simulink model "Speed_Controller_Test_forTD"  (Simulink 6.6)
settings: Solver=ode4  SolverMode=SingleTasking  StartTime=0.0  StopTime=252  FixedStep=0.01  RelTol=1e-3
InitFcn:
  | tempomat_para
StopFcn:
  | clear;
values from neighbouring files (symbols this model uses):
  A = 1.9    [tempomat_para.m]
  a_Fzg_max = 2    [tempomat_para.m]
  a_Fzg_min = -2    [tempomat_para.m]
  cw = 0.32    [tempomat_para.m]
  gang = [1 2 3 4]    [tempomat_para.m]
  gang_vec = [1 2 3 4]    [tempomat_para.m]
  i_anteil = 5    [tempomat_para.m]
  i_d = 3.42    [tempomat_para.m]
  i_g = [3.91 2.17 1.37 1.00]    [tempomat_para.m]
  lambda_gang = [1.3 1.25  1.17  1.05]    [tempomat_para.m]
  m_Fzg = 1400    [tempomat_para.m]
  M_mot_max = [130 149 163 170 168 166 162 158 150 139 123 80]    [tempomat_para.m]
  M_mot_min = [0 -40]    [tempomat_para.m]
  n_mot0 = 1000    [tempomat_para.m]
  n_mot_max = 1000:500:6500    [tempomat_para.m]
  n_mot_min = [1000 6500]    [tempomat_para.m]
  p_anteil = 100    [tempomat_para.m]
  r_dyn = 0.28    [tempomat_para.m]
  rho = 1.202    [tempomat_para.m]
  t_sch = 0.2    [tempomat_para.m]
  TI = [block '/TI']    [PSTI_callback.m]
  v_Fzg_ms0 = 0    [tempomat_para.m]
undefined symbols (not defined in the file or in its folder): Drossel_mat, getdatatypespecs
libraries: simulink x116, fzgbib x3
(part 9 of 9)

== system Speed_Controller_Test_forTD/Validation and  Test Evaluation/R1 Speed Control step response/Complete step & CC active + no target & Speed Control active/Complete step detection/Step detection/Active if signals constant for some specified time/Time since signal constant1/Detect constant ==
  Signal : Inport
  Clock : Clock
      settings: Decimation=10
  Constant1 : Constant  Value=0  OutDataTypeMode=boolean
  Memory : Memory
  Relative tolerance : Subsystem
  Switch : Switch  Criteria=u2 > Threshold
  Constant : Outport
  wires:
  Signal/1 -> Relative tolerance/1(sig), Memory/1
  Memory/1 -> Relative tolerance/2(ref)
  Constant1/1 -> Switch/3
  Clock/1 -> Switch/2
  Relative tolerance/1(sig == ref) -> Switch/1
  Switch/1 -> Constant/1

== system Speed_Controller_Test_forTD/Validation and  Test Evaluation/R1 Speed Control step response/Complete step & CC active + no target & Speed Control active/Complete step detection/Step detection reset/Active if signals constant for some specified time/Time since signal constant/Detect constant ==
  Signal : Inport
  Clock : Clock
      settings: Decimation=10
  Constant1 : Constant  Value=0  OutDataTypeMode=boolean
  Memory : Memory
  Relative tolerance : Subsystem
  Switch : Switch  Criteria=u2 > Threshold
  Constant : Outport
  wires:
  Signal/1 -> Memory/1, Relative tolerance/1(sig)
  Memory/1 -> Relative tolerance/2(ref)
  Constant1/1 -> Switch/3
  Clock/1 -> Switch/2
  Relative tolerance/1(sig == ref) -> Switch/1
  Switch/1 -> Constant/1

== system Speed_Controller_Test_forTD/Validation and  Test Evaluation/R1 Speed Control step response/Complete step & CC active + no target & Speed Control active/Complete step detection/Step detection reset/Active if signals constant for some specified time/Time since signal constant1/Detect constant ==
  Signal : Inport
  Clock : Clock
      settings: Decimation=10
  Constant1 : Constant  Value=0  OutDataTypeMode=boolean
  Memory : Memory
  Relative tolerance : Subsystem
  Switch : Switch  Criteria=u2 > Threshold
  Constant : Outport
  wires:
  Switch/1 -> Constant/1
  Relative tolerance/1(sig == ref) -> Switch/1
  Clock/1 -> Switch/2
  Constant1/1 -> Switch/3
  Memory/1 -> Relative tolerance/2(ref)
  Signal/1 -> Memory/1, Relative tolerance/1(sig)

== system Speed_Controller_Test_forTD/Validation and  Test Evaluation/R1 Speed Control step response/Maximum overshoot < 5 &  Steady state error < 5/Step response characteristics/Step response characteristics extraction/Extract maximum overshoot/Active if signals constant for some specified time/Time since signal constant ==
  Signal : Inport
  Clock : Clock
      settings: Decimation=10
  Detect constant : Subsystem  TreatAsAtomicUnit=on  mask(Feature extraction block){RT=0.0001}
      mask prompts: RT "Relative tolerance in %"
      mask help: Detect if the signal value is constant (using the last two signal values) allowing for a user-defined relative deviation
      mask CallbackString:
      | if or( (str2double(get_param(gcb,'RT')) < 0), (str2double(get_param(gcb,'RT')) > 100))
      |     error(['Relative tolerance value (' get_param(gcb,'RT') ') out of range. Please give a value between 0 and 100.']);
      | else
      |     set_param([gcb '/Relative tolerance/Relative Tolerance'],'Value',get_param(gcb,'RT'));
      | end
  Logical Operator : Logic  Operator=NAND  AllPortsSameDT=off  OutDataTypeMode=Boolean
  Logical Operator1 : Logic  Operator=NOT  AllPortsSameDT=off  OutDataTypeMode=Boolean
  Memory : Memory  Orientation=left
  Memory1 : Memory
  Subtract : Sum  Inputs=-+  OutScaling=2^-10
  Switch : Switch  Criteria=u2 > Threshold
  Trigger : Outport
  Feature : Outport  Port=2
  wires:
  Signal/1 -> Detect constant/1(Signal)
  Detect constant/1(Constant) -> Trigger/1, Logical Operator/1, Memory1/1
  Subtract/1 -> Feature/1
  Clock/1 -> Subtract/2, Switch/3
  Switch/1 -> Subtract/1, Memory/1
  Memory/1 -> Switch/1
  Memory1/1 -> Logical Operator1/1
  Logical Operator1/1 -> Logical Operator/2
  Logical Operator/1 -> Switch/2

== system Speed_Controller_Test_forTD/Validation and  Test Evaluation/R1 Speed Control step response/Maximum overshoot < 5 &  Steady state error < 5/Step response characteristics/Step response characteristics extraction/Extract maximum overshoot/Active if signals constant for some specified time/Time since signal constant1 ==
  Signal : Inport
  Clock : Clock
      settings: Decimation=10
  Detect constant : Subsystem  TreatAsAtomicUnit=on  mask(Feature extraction block){RT=0.0001}
      mask prompts: RT "Relative tolerance in %"
      mask help: Detect if the signal value is constant (using the last two signal values) allowing for a user-defined relative deviation
      mask CallbackString:
      | if or( (str2double(get_param(gcb,'RT')) < 0), (str2double(get_param(gcb,'RT')) > 100))
      |     error(['Relative tolerance value (' get_param(gcb,'RT') ') out of range. Please give a value between 0 and 100.']);
      | else
      |     set_param([gcb '/Relative tolerance/Relative Tolerance'],'Value',get_param(gcb,'RT'));
      | end
  Logical Operator : Logic  Operator=NAND  AllPortsSameDT=off  OutDataTypeMode=Boolean
  Logical Operator1 : Logic  Operator=NOT  AllPortsSameDT=off  OutDataTypeMode=Boolean
  Memory : Memory  Orientation=left
  Memory1 : Memory
  Subtract : Sum  Inputs=-+  OutScaling=2^-10
  Switch : Switch  Criteria=u2 > Threshold
  Trigger : Outport
  Feature : Outport  Port=2
  wires:
  Logical Operator/1 -> Switch/2
  Logical Operator1/1 -> Logical Operator/2
  Memory1/1 -> Logical Operator1/1
  Memory/1 -> Switch/1
  Switch/1 -> Memory/1, Subtract/1
  Clock/1 -> Switch/3, Subtract/2
  Subtract/1 -> Feature/1
  Detect constant/1(Constant) -> Memory1/1, Logical Operator/1, Trigger/1
  Signal/1 -> Detect constant/1(Signal)

== system Speed_Controller_Test_forTD/Validation and  Test Evaluation/R1 Speed Control step response/Maximum overshoot < 5 &  Steady state error < 5/Step response characteristics/Step response characteristics extraction/Extract maximum overshoot/Hold value with counter/Execution counter ==
  Reset : Inport
  Add1 : Sum  OutScaling=2^-10
  Constant : Constant
  Logical Operator : Logic  Operator=NOT  AllPortsSameDT=off  OutDataTypeMode=Specify via dialog
  Memory : Memory  Orientation=left  InheritSampleTime=on
  Product : Product  RndMeth=Zero
  Counter : Outport
  wires:
  Product/1 -> Counter/1, Memory/1
  Logical Operator/1 -> Product/1
  Add1/1 -> Product/2
  Constant/1 -> Add1/1
  Reset/1 -> Logical Operator/1
  Memory/1 -> Add1/2

== system Speed_Controller_Test_forTD/Validation and  Test Evaluation/R1 Speed Control step response/Maximum overshoot < 5 &  Steady state error < 5/Step response characteristics/Step response characteristics extraction/Extract maximum overshoot/Step response moving average and initial conditions before step/Flip if new step ==
  Enable : EnablePort
  Logical Operator : Logic  Operator=NOT  AllPortsSameDT=off  OutDataTypeMode=Boolean
  Memory : Memory  Orientation=left
  0/1 : Outport
  wires:
  Memory/1 -> Logical Operator/1
  Logical Operator/1 -> 0/1/1, Memory/1

== system Speed_Controller_Test_forTD/Validation and  Test Evaluation/R1 Speed Control step response/Maximum overshoot < 5 &  Steady state error < 5/Step response characteristics/Step response characteristics extraction/Extract maximum overshoot/Trigger hold value/Negative step ==
  u : Inport
  Compare : RelationalOperator  Operator=>  LogicOutDataTypeMode=Specify via dialog  ZeroCross=off  InputSameDT=on
  Ground : Ground
  y : Outport
  wires:
  Compare/1 -> y/1
  Ground/1 -> Compare/2
  u/1 -> Compare/1

== system Speed_Controller_Test_forTD/Validation and  Test Evaluation/R1 Speed Control step response/Maximum overshoot < 5 &  Steady state error < 5/Step response characteristics/Step response characteristics extraction/Extract maximum overshoot/Trigger hold value/Positive step ==
  u : Inport
  Compare : RelationalOperator  Operator=<  LogicOutDataTypeMode=Specify via dialog  ZeroCross=off  InputSameDT=on
  Ground : Ground
  y : Outport
  wires:
  Compare/1 -> y/1
  Ground/1 -> Compare/2
  u/1 -> Compare/1

== system Speed_Controller_Test_forTD/Validation and  Test Evaluation/R1 Speed Control step response/Maximum overshoot < 5 &  Steady state error < 5/Step response characteristics/Step response characteristics extraction/Extract rise time/Time difference/Execution counter ==
  Reset : Inport
  Add1 : Sum  OutScaling=2^-10
  Constant : Constant
  Logical Operator : Logic  Operator=NOT  AllPortsSameDT=off  OutDataTypeMode=Specify via dialog
  Memory : Memory  Orientation=left  InheritSampleTime=on
  Product : Product  RndMeth=Zero
  Counter : Outport
  wires:
  Product/1 -> Counter/1, Memory/1
  Logical Operator/1 -> Product/1
  Add1/1 -> Product/2
  Constant/1 -> Add1/1
  Reset/1 -> Logical Operator/1
  Memory/1 -> Add1/2

== system Speed_Controller_Test_forTD/Validation and  Test Evaluation/R1 Speed Control step response/Maximum overshoot < 5 &  Steady state error < 5/Step response characteristics/Step response reset/Active if signals constant for some specified time/Time since signal constant/Detect constant ==
  Signal : Inport
  Clock : Clock
      settings: Decimation=10
  Constant1 : Constant  Value=0  OutDataTypeMode=boolean
  Memory : Memory
  Relative tolerance : Subsystem
  Switch : Switch  Criteria=u2 > Threshold
  Constant : Outport
  wires:
  Signal/1 -> Memory/1, Relative tolerance/1(sig)
  Memory/1 -> Relative tolerance/2(ref)
  Constant1/1 -> Switch/3
  Clock/1 -> Switch/2
  Relative tolerance/1(sig == ref) -> Switch/1
  Switch/1 -> Constant/1

== system Speed_Controller_Test_forTD/Validation and  Test Evaluation/R1 Speed Control step response/Maximum overshoot < 5 &  Steady state error < 5/Step response characteristics/Step response reset/Active if signals constant for some specified time/Time since signal constant1/Detect constant ==
  Signal : Inport
  Clock : Clock
      settings: Decimation=10
  Constant1 : Constant  Value=0  OutDataTypeMode=boolean
  Memory : Memory
  Relative tolerance : Subsystem
  Switch : Switch  Criteria=u2 > Threshold
  Constant : Outport
  wires:
  Switch/1 -> Constant/1
  Relative tolerance/1(sig == ref) -> Switch/1
  Clock/1 -> Switch/2
  Constant1/1 -> Switch/3
  Memory/1 -> Relative tolerance/2(ref)
  Signal/1 -> Memory/1, Relative tolerance/1(sig)

== system Speed_Controller_Test_forTD/Validation and  Test Evaluation/R1 Speed Control step response/Maximum overshoot < 5 &  Steady state error < 5/Step response characteristics/Step response trigger/Active if signals constant for some specified time/Time since signal constant/Detect constant ==
  Signal : Inport
  Clock : Clock
      settings: Decimation=10
  Constant1 : Constant  Value=0  OutDataTypeMode=boolean
  Memory : Memory
  Relative tolerance : Subsystem
  Switch : Switch  Criteria=u2 > Threshold
  Constant : Outport
  wires:
  Signal/1 -> Memory/1, Relative tolerance/1(sig)
  Memory/1 -> Relative tolerance/2(ref)
  Constant1/1 -> Switch/3
  Clock/1 -> Switch/2
  Relative tolerance/1(sig == ref) -> Switch/1
  Switch/1 -> Constant/1

== system Speed_Controller_Test_forTD/Validation and  Test Evaluation/R1 Speed Control step response/Maximum overshoot < 5 &  Steady state error < 5/Step response characteristics/Step response trigger/Active if signals constant for some specified time/Time since signal constant1/Detect constant ==
  Signal : Inport
  Clock : Clock
      settings: Decimation=10
  Constant1 : Constant  Value=0  OutDataTypeMode=boolean
  Memory : Memory
  Relative tolerance : Subsystem
  Switch : Switch  Criteria=u2 > Threshold
  Constant : Outport
  wires:
  Switch/1 -> Constant/1
  Relative tolerance/1(sig == ref) -> Switch/1
  Clock/1 -> Switch/2
  Constant1/1 -> Switch/3
  Memory/1 -> Relative tolerance/2(ref)
  Signal/1 -> Memory/1, Relative tolerance/1(sig)

== system Speed_Controller_Test_forTD/Validation and  Test Evaluation/R2 Speed Control velocity restoration time after simple  acceleration/deceleration/CC active + no target & Speed Control active & step of V_Des = |1|  with time periods >= 7s/Step with step size=|1|  and time periods >= 6s detection/Step detection/Active if signals constant for some specified time/Time since signal constant1/Detect constant ==
  Signal : Inport
  Clock : Clock
      settings: Decimation=10
  Constant1 : Constant  Value=0  OutDataTypeMode=boolean
  Memory : Memory
  Relative tolerance : Subsystem
  Switch : Switch  Criteria=u2 > Threshold
  Constant : Outport
  wires:
  Switch/1 -> Constant/1
  Relative tolerance/1(sig == ref) -> Switch/1
  Clock/1 -> Switch/2
  Constant1/1 -> Switch/3
  Memory/1 -> Relative tolerance/2(ref)
  Signal/1 -> Memory/1, Relative tolerance/1(sig)

== system Speed_Controller_Test_forTD/Validation and  Test Evaluation/R1 Speed Control step response/Complete step & CC active + no target & Speed Control active/Complete step detection/Step detection/Active if signals constant for some specified time/Time since signal constant/Detect constant/Relative tolerance ==
  sig : Inport
  ref : Inport  Port=2
  Abs : Abs
  Abs1 : Abs
  Add : Sum  Inputs=+-  OutScaling=2^-10
  Divide1 : Product  Inputs=**/  OutScaling=2^-10
  Max : Constant  Value=100
  Relational Operator : RelationalOperator  Operator=<=  LogicOutDataTypeMode=Boolean
  Relative Tolerance : Constant  Value=0.001
  sig == ref : Outport
  wires:
  Abs1/1 -> Divide1/1
  Relational Operator/1 -> sig == ref/1
  Relative Tolerance/1 -> Divide1/2
  Max/1 -> Divide1/3
  Divide1/1 -> Relational Operator/2
  ref/1 -> Abs1/1, Add/2
  sig/1 -> Add/1
  Add/1 -> Abs/1
  Abs/1 -> Relational Operator/1

== system Speed_Controller_Test_forTD/Validation and  Test Evaluation/R1 Speed Control step response/Complete step & CC active + no target & Speed Control active/Complete step detection/Step detection/Active if signals constant for some specified time/Time since signal constant1/Detect constant/Relative tolerance ==
  sig : Inport
  ref : Inport  Port=2
  Abs : Abs
  Abs1 : Abs
  Add : Sum  Inputs=+-  OutScaling=2^-10
  Divide1 : Product  Inputs=**/  OutScaling=2^-10
  Max : Constant  Value=100
  Relational Operator : RelationalOperator  Operator=<=  LogicOutDataTypeMode=Boolean
  Relative Tolerance : Constant  Value=0.001
  sig == ref : Outport
  wires:
  Abs1/1 -> Divide1/1
  Relational Operator/1 -> sig == ref/1
  Relative Tolerance/1 -> Divide1/2
  Max/1 -> Divide1/3
  Divide1/1 -> Relational Operator/2
  ref/1 -> Abs1/1, Add/2
  sig/1 -> Add/1
  Add/1 -> Abs/1
  Abs/1 -> Relational Operator/1

== system Speed_Controller_Test_forTD/Validation and  Test Evaluation/R1 Speed Control step response/Complete step & CC active + no target & Speed Control active/Complete step detection/Step detection reset/Active if signals constant for some specified time/Time since signal constant/Detect constant/Relative tolerance ==
  sig : Inport
  ref : Inport  Port=2
  Abs : Abs
  Abs1 : Abs
  Add : Sum  Inputs=+-  OutScaling=2^-10
  Divide1 : Product  Inputs=**/  OutScaling=2^-10
  Max : Constant  Value=100
  Relational Operator : RelationalOperator  Operator=<=  LogicOutDataTypeMode=Boolean
  Relative Tolerance : Constant  Value=0.0001
  sig == ref : Outport
  wires:
  Abs/1 -> Relational Operator/1
  Add/1 -> Abs/1
  sig/1 -> Add/1
  ref/1 -> Add/2, Abs1/1
  Divide1/1 -> Relational Operator/2
  Max/1 -> Divide1/3
  Relative Tolerance/1 -> Divide1/2
  Relational Operator/1 -> sig == ref/1
  Abs1/1 -> Divide1/1

== system Speed_Controller_Test_forTD/Validation and  Test Evaluation/R1 Speed Control step response/Complete step & CC active + no target & Speed Control active/Complete step detection/Step detection reset/Active if signals constant for some specified time/Time since signal constant1/Detect constant/Relative tolerance ==
  sig : Inport
  ref : Inport  Port=2
  Abs : Abs
  Abs1 : Abs
  Add : Sum  Inputs=+-  OutScaling=2^-10
  Divide1 : Product  Inputs=**/  OutScaling=2^-10
  Max : Constant  Value=100
  Relational Operator : RelationalOperator  Operator=<=  LogicOutDataTypeMode=Boolean
  Relative Tolerance : Constant  Value=0.0001
  sig == ref : Outport
  wires:
  Abs/1 -> Relational Operator/1
  Add/1 -> Abs/1
  sig/1 -> Add/1
  ref/1 -> Add/2, Abs1/1
  Divide1/1 -> Relational Operator/2
  Max/1 -> Divide1/3
  Relative Tolerance/1 -> Divide1/2
  Relational Operator/1 -> sig == ref/1
  Abs1/1 -> Divide1/1

== system Speed_Controller_Test_forTD/Validation and  Test Evaluation/R1 Speed Control step response/Maximum overshoot < 5 &  Steady state error < 5/Step response characteristics/Step response characteristics extraction/Extract maximum overshoot/Active if signals constant for some specified time/Time since signal constant/Detect constant ==
  Signal : Inport
  Clock : Clock
      settings: Decimation=10
  Constant1 : Constant  Value=0  OutDataTypeMode=boolean
  Memory : Memory
  Relative tolerance : Subsystem
  Switch : Switch  Criteria=u2 > Threshold
  Constant : Outport
  wires:
  Signal/1 -> Memory/1, Relative tolerance/1(sig)
  Memory/1 -> Relative tolerance/2(ref)
  Constant1/1 -> Switch/3
  Clock/1 -> Switch/2
  Relative tolerance/1(sig == ref) -> Switch/1
  Switch/1 -> Constant/1

== system Speed_Controller_Test_forTD/Validation and  Test Evaluation/R1 Speed Control step response/Maximum overshoot < 5 &  Steady state error < 5/Step response characteristics/Step response characteristics extraction/Extract maximum overshoot/Active if signals constant for some specified time/Time since signal constant1/Detect constant ==
  Signal : Inport
  Clock : Clock
      settings: Decimation=10
  Constant1 : Constant  Value=0  OutDataTypeMode=boolean
  Memory : Memory
  Relative tolerance : Subsystem
  Switch : Switch  Criteria=u2 > Threshold
  Constant : Outport
  wires:
  Switch/1 -> Constant/1
  Relative tolerance/1(sig == ref) -> Switch/1
  Clock/1 -> Switch/2
  Constant1/1 -> Switch/3
  Memory/1 -> Relative tolerance/2(ref)
  Signal/1 -> Memory/1, Relative tolerance/1(sig)

== system Speed_Controller_Test_forTD/Validation and  Test Evaluation/R1 Speed Control step response/Maximum overshoot < 5 &  Steady state error < 5/Step response characteristics/Step response reset/Active if signals constant for some specified time/Time since signal constant/Detect constant/Relative tolerance ==
  sig : Inport
  ref : Inport  Port=2
  Abs : Abs
  Abs1 : Abs
  Add : Sum  Inputs=+-  OutScaling=2^-10
  Divide1 : Product  Inputs=**/  OutScaling=2^-10
  Max : Constant  Value=100
  Relational Operator : RelationalOperator  Operator=<=  LogicOutDataTypeMode=Boolean
  Relative Tolerance : Constant  Value=0.0001
  sig == ref : Outport
  wires:
  Abs/1 -> Relational Operator/1
  Add/1 -> Abs/1
  sig/1 -> Add/1
  ref/1 -> Add/2, Abs1/1
  Divide1/1 -> Relational Operator/2
  Max/1 -> Divide1/3
  Relative Tolerance/1 -> Divide1/2
  Relational Operator/1 -> sig == ref/1
  Abs1/1 -> Divide1/1

== system Speed_Controller_Test_forTD/Validation and  Test Evaluation/R1 Speed Control step response/Maximum overshoot < 5 &  Steady state error < 5/Step response characteristics/Step response reset/Active if signals constant for some specified time/Time since signal constant1/Detect constant/Relative tolerance ==
  sig : Inport
  ref : Inport  Port=2
  Abs : Abs
  Abs1 : Abs
  Add : Sum  Inputs=+-  OutScaling=2^-10
  Divide1 : Product  Inputs=**/  OutScaling=2^-10
  Max : Constant  Value=100
  Relational Operator : RelationalOperator  Operator=<=  LogicOutDataTypeMode=Boolean
  Relative Tolerance : Constant  Value=0.0001
  sig == ref : Outport
  wires:
  Abs/1 -> Relational Operator/1
  Add/1 -> Abs/1
  sig/1 -> Add/1
  ref/1 -> Add/2, Abs1/1
  Divide1/1 -> Relational Operator/2
  Max/1 -> Divide1/3
  Relative Tolerance/1 -> Divide1/2
  Relational Operator/1 -> sig == ref/1
  Abs1/1 -> Divide1/1

== system Speed_Controller_Test_forTD/Validation and  Test Evaluation/R1 Speed Control step response/Maximum overshoot < 5 &  Steady state error < 5/Step response characteristics/Step response trigger/Active if signals constant for some specified time/Time since signal constant/Detect constant/Relative tolerance ==
  sig : Inport
  ref : Inport  Port=2
  Abs : Abs
  Abs1 : Abs
  Add : Sum  Inputs=+-  OutScaling=2^-10
  Divide1 : Product  Inputs=**/  OutScaling=2^-10
  Max : Constant  Value=100
  Relational Operator : RelationalOperator  Operator=<=  LogicOutDataTypeMode=Boolean
  Relative Tolerance : Constant  Value=0.0001
  sig == ref : Outport
  wires:
  Abs/1 -> Relational Operator/1
  Add/1 -> Abs/1
  sig/1 -> Add/1
  ref/1 -> Add/2, Abs1/1
  Divide1/1 -> Relational Operator/2
  Max/1 -> Divide1/3
  Relative Tolerance/1 -> Divide1/2
  Relational Operator/1 -> sig == ref/1
  Abs1/1 -> Divide1/1

== system Speed_Controller_Test_forTD/Validation and  Test Evaluation/R1 Speed Control step response/Maximum overshoot < 5 &  Steady state error < 5/Step response characteristics/Step response trigger/Active if signals constant for some specified time/Time since signal constant1/Detect constant/Relative tolerance ==
  sig : Inport
  ref : Inport  Port=2
  Abs : Abs
  Abs1 : Abs
  Add : Sum  Inputs=+-  OutScaling=2^-10
  Divide1 : Product  Inputs=**/  OutScaling=2^-10
  Max : Constant  Value=100
  Relational Operator : RelationalOperator  Operator=<=  LogicOutDataTypeMode=Boolean
  Relative Tolerance : Constant  Value=0.0001
  sig == ref : Outport
  wires:
  Abs/1 -> Relational Operator/1
  Add/1 -> Abs/1
  sig/1 -> Add/1
  ref/1 -> Add/2, Abs1/1
  Divide1/1 -> Relational Operator/2
  Max/1 -> Divide1/3
  Relative Tolerance/1 -> Divide1/2
  Relational Operator/1 -> sig == ref/1
  Abs1/1 -> Divide1/1

== system Speed_Controller_Test_forTD/Validation and  Test Evaluation/R2 Speed Control velocity restoration time after simple  acceleration/deceleration/CC active + no target & Speed Control active & step of V_Des = |1|  with time periods >= 7s/Step with step size=|1|  and time periods >= 6s detection/Step detection/Active if signals constant for some specified time/Time since signal constant1/Detect constant/Relative tolerance ==
  sig : Inport
  ref : Inport  Port=2
  Abs : Abs
  Abs1 : Abs
  Add : Sum  Inputs=+-  OutScaling=2^-10
  Divide1 : Product  Inputs=**/  OutScaling=2^-10
  Max : Constant  Value=100
  Relational Operator : RelationalOperator  Operator=<=  LogicOutDataTypeMode=Boolean
  Relative Tolerance : Constant  Value=0.0001
  sig == ref : Outport
  wires:
  Abs/1 -> Relational Operator/1
  Add/1 -> Abs/1
  sig/1 -> Add/1
  ref/1 -> Add/2, Abs1/1
  Divide1/1 -> Relational Operator/2
  Max/1 -> Divide1/3
  Relative Tolerance/1 -> Divide1/2
  Relational Operator/1 -> sig == ref/1
  Abs1/1 -> Divide1/1

== system Speed_Controller_Test_forTD/Validation and  Test Evaluation/R1 Speed Control step response/Maximum overshoot < 5 &  Steady state error < 5/Step response characteristics/Step response characteristics extraction/Extract maximum overshoot/Active if signals constant for some specified time/Time since signal constant/Detect constant/Relative tolerance ==
  sig : Inport
  ref : Inport  Port=2
  Abs : Abs
  Abs1 : Abs
  Add : Sum  Inputs=+-  OutScaling=2^-10
  Divide1 : Product  Inputs=**/  OutScaling=2^-10
  Max : Constant  Value=100
  Relational Operator : RelationalOperator  Operator=<=  LogicOutDataTypeMode=Boolean
  Relative Tolerance : Constant  Value=0.0001
  sig == ref : Outport
  wires:
  Abs/1 -> Relational Operator/1
  Add/1 -> Abs/1
  sig/1 -> Add/1
  ref/1 -> Add/2, Abs1/1
  Divide1/1 -> Relational Operator/2
  Max/1 -> Divide1/3
  Relative Tolerance/1 -> Divide1/2
  Relational Operator/1 -> sig == ref/1
  Abs1/1 -> Divide1/1

== system Speed_Controller_Test_forTD/Validation and  Test Evaluation/R1 Speed Control step response/Maximum overshoot < 5 &  Steady state error < 5/Step response characteristics/Step response characteristics extraction/Extract maximum overshoot/Active if signals constant for some specified time/Time since signal constant1/Detect constant/Relative tolerance ==
  sig : Inport
  ref : Inport  Port=2
  Abs : Abs
  Abs1 : Abs
  Add : Sum  Inputs=+-  OutScaling=2^-10
  Divide1 : Product  Inputs=**/  OutScaling=2^-10
  Max : Constant  Value=100
  Relational Operator : RelationalOperator  Operator=<=  LogicOutDataTypeMode=Boolean
  Relative Tolerance : Constant  Value=0.0001
  sig == ref : Outport
  wires:
  Abs/1 -> Relational Operator/1
  Add/1 -> Abs/1
  sig/1 -> Add/1
  ref/1 -> Add/2, Abs1/1
  Divide1/1 -> Relational Operator/2
  Max/1 -> Divide1/3
  Relative Tolerance/1 -> Divide1/2
  Relational Operator/1 -> sig == ref/1
  Abs1/1 -> Divide1/1
